simulink model "simulation"  (R2024b)
settings: Solver=ode4  StartTime=0.0  StopTime=100  FixedStep=0.01  RelTol=1e-3
values from neighbouring files (symbols this model uses):
  Eta_initial = [0;0;0]    [Feb21_tutorial.m]    (also in model.m; tutorial.m)
  mass = 18    [Feb21_tutorial.m]
  matrix_Mass = rigid_body_Mass + added_Mass    [Feb21_tutorial.m]
  N_coef_d33_over_r = N_coef_d33(1:3)    [Feb21_tutorial.m]
  V_initial = [0;0;0]    [Feb21_tutorial.m]    (also in model.m = [0;0;0]+[EN.current_speed';0]; tutorial.m)
  X_coef_d11_over_u = X_coef_d11(1:3)    [Feb21_tutorial.m]
  x_u_dot = 1.2    [Feb21_tutorial.m]
  Y_coef_d22_over_v = Y_coef_d22(1:3)    [Feb21_tutorial.m]
  y_v_dot = 66.1    [Feb21_tutorial.m]
undefined symbols (not defined in the file or in its folder): Cm, Jm
settings Model: Creator=Irene  LastModifiedBy=Santiago

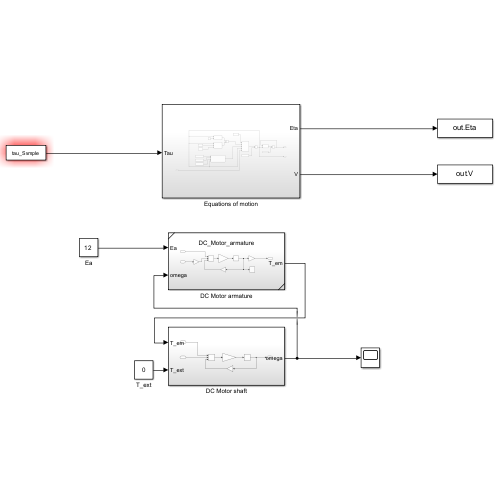
[thumbnail: Simulink's stored preview of the top-level diagram]
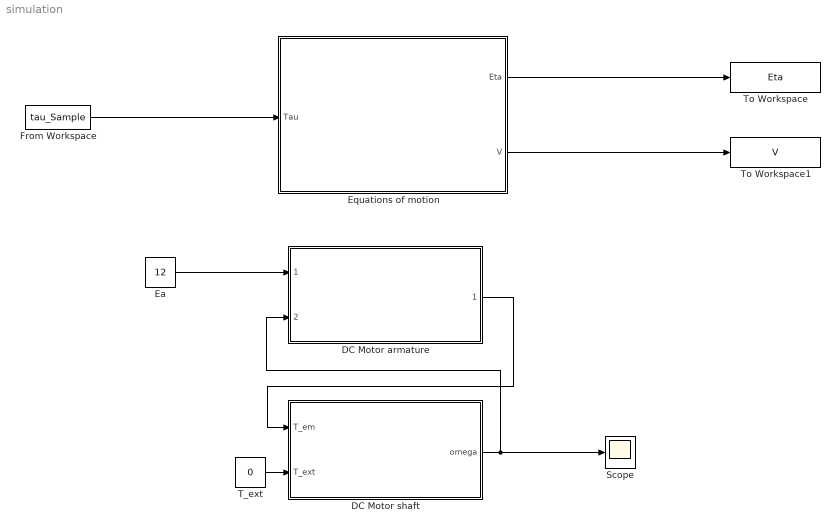
== system simulation ==
  DC Motor armature : Subsystem  ReferencedSubsystem=DC_Motor_armature
  DC Motor shaft : Subsystem
  Ea : Constant  Value=12
  Equations of motion : Subsystem
  From Workspace : FromWorkspace  VariableName=tau_Sample
  Scope : Scope
  T_ext : Constant  Value=0
  To Workspace : ToWorkspace  VariableName=Eta  SampleTime=-1
  To Workspace1 : ToWorkspace  VariableName=V  SampleTime=-1
  wires:
  From Workspace/1 -> Equations of motion/1(Tau)
  Equations of motion/1(Eta) -> To Workspace/1
  Equations of motion/2(V) -> To Workspace1/1
  Ea/1 -> DC Motor armature/1
  DC Motor shaft/1(omega) -> Scope/1, DC Motor armature/2
  DC Motor armature/1 -> DC Motor shaft/1(T_em)
  T_ext/1 -> DC Motor shaft/2(T_ext)

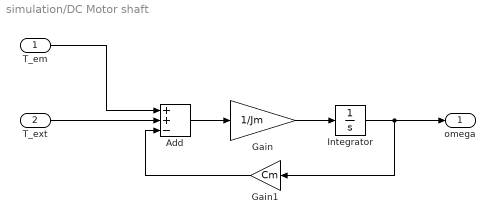
== system simulation/DC Motor shaft ==
  T_em : Inport
  T_ext : Inport  Port=2
  Add : Sum  Inputs=++-
  Gain : Gain  Gain=1/Jm
  Gain1 : Gain  Gain=Cm
  Integrator : Integrator
  omega : Outport
  wires:
  Gain/1 -> Integrator/1
  Add/1 -> Gain/1
  Integrator/1 -> omega/1, Gain1/1
  Gain1/1 -> Add/3
  T_em/1 -> Add/1
  T_ext/1 -> Add/2

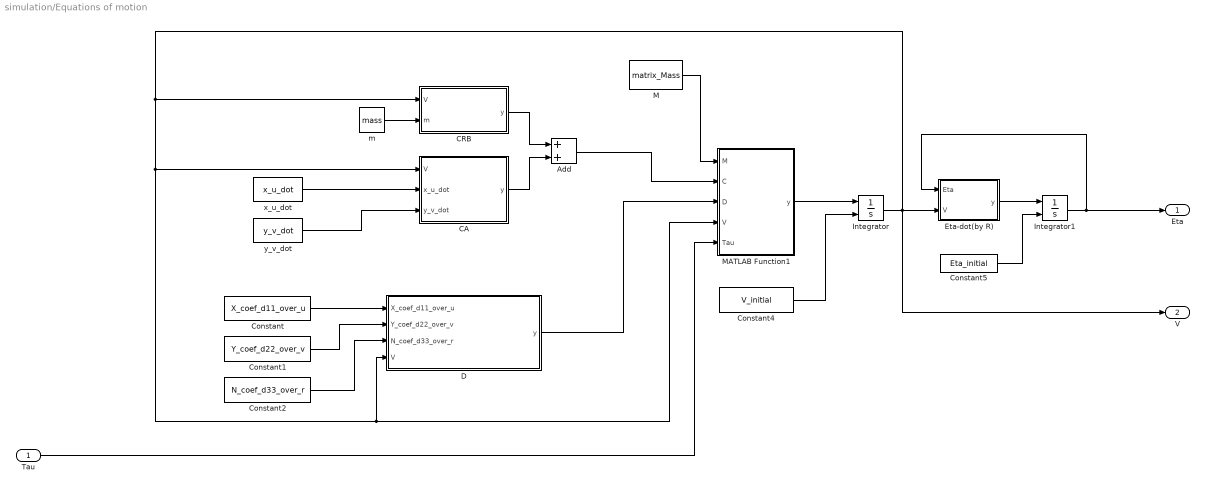
== system simulation/Equations of motion ==
  Tau : Inport
  Add : Sum
  CA : MATLAB Function  TreatAsAtomicUnit=on
  CRB : MATLAB Function  TreatAsAtomicUnit=on
  Constant : Constant  Value=X_coef_d11_over_u
  Constant1 : Constant  Value=Y_coef_d22_over_v
  Constant2 : Constant  Value=N_coef_d33_over_r
  Constant4 : Constant  Value=V_initial
  Constant5 : Constant  Value=Eta_initial
  D : MATLAB Function  TreatAsAtomicUnit=on
  Eta-dot(by R) : MATLAB Function  TreatAsAtomicUnit=on
  Integrator : Integrator  InitialConditionSource=external
  Integrator1 : Integrator  InitialConditionSource=external
  M : Constant  Value=matrix_Mass
  MATLAB Function1 : MATLAB Function  TreatAsAtomicUnit=on
  m : Constant  Value=mass
  "x_u_dot " : Constant  Value=x_u_dot
  y_v_dot : Constant  Value=y_v_dot
  Eta : Outport
  V : Outport  Port=2
  wires:
  Constant1/1 -> D/2(Y_coef_d22_over_v)
  m/1 -> CRB/2(m)
  Constant4/1 -> Integrator/2
  Integrator1/1 -> Eta/1, Eta-dot(by R)/1(Eta)
  "x_u_dot "/1 -> CA/2(x_u_dot)
  Integrator/1 -> V/1, Eta-dot(by R)/2(V), MATLAB Function1/4(V), D/4(V), CA/1(V), CRB/1(V)
  MATLAB Function1/1(y) -> Integrator/1
  Constant2/1 -> D/3(N_coef_d33_over_r)
  y_v_dot/1 -> CA/3(y_v_dot)
  Add/1 -> MATLAB Function1/2(C)
  Constant5/1 -> Integrator1/2
  D/1(y) -> MATLAB Function1/3(D)
  CA/1(y) -> Add/2
  Eta-dot(by R)/1(y) -> Integrator1/1
  M/1 -> MATLAB Function1/1(M)
  CRB/1(y) -> Add/1
  Constant/1 -> D/1(X_coef_d11_over_u)
  Tau/1 -> MATLAB Function1/5(Tau)

== matlab function simulation/Equations of motion/CA ==
  data: V input; y output; x_u_dot input; y_v_dot input
function y = C_A(V,x_u_dot,y_v_dot)
a1=x_u_dot*V(1);
a2=y_v_dot*V(2);
y = [0   0   a2;
     0   0  -a1;
     -a2 a1  0];

== matlab function simulation/Equations of motion/CRB ==
  data: V input; y output; m input
function y = C_RB(V,m)

y = [0       0      -m*V(2);
     0       0      m*V(1) ;
     m*V(2) -m*V(1) 0     ];

== matlab function simulation/Equations of motion/MATLAB Function1 ==
  data: M input; C input; D input; V input; Tau input; y output
function y = motion_V_dot(M,C,D,V,Tau)

y = inv(M)*(Tau-C*V-D*V);

== matlab function simulation/Equations of motion/D ==
  data: X_coef_d11_over_u input; y output; Y_coef_d22_over_v input; N_coef_d33_over_r input; V input
function y = D(X_coef_d11_over_u,Y_coef_d22_over_v,N_coef_d33_over_r,V)
d11=polyval(X_coef_d11_over_u,V(1));
d22=polyval(Y_coef_d22_over_v,V(2));
d33=polyval(N_coef_d33_over_r,V(3));
y = diag([d11 d22 d33]);

== matlab function simulation/Equations of motion/Eta-dot(by R) ==
  data: Eta input; y output; V input
function y = Eta_dot(Eta,V)
psi=Eta(3);
R = [cos(psi) -sin(psi) 0;
     sin(psi)  cos(psi) 0;
      0        0        1];
y=R*V;
